simulink model "Australian14gen_following_inertia"  (R2017b)
settings: Solver=ode23tb  StartTime=0.0  StopTime=30  FixedStep=1e-3  RelTol=1e-5  AbsTol=1e-3  EnableMultiTasking=on
PreLoadFcn:
  | dataaustralian14gen
values from neighbouring files (symbols this model uses):
  alpha = -sys.follin.opt.alpha*1e8    [main_following.m]    (also in optimgains.mat = [-2447350365.29 -12566370614.4 -12566370614.4 -11730281347.7)
  bus_v = [ 101	15 ... (first row only)    [dataaustralian14gen.m]
  comp = [ 1	211	0	0 ... (first row only)    [dataaustralian14gen.m]
  dist = sys.follin.dist    [main_following.m]    (also in main_forming.m = sys.formin.dist)
  Exc = [ 101	0	 200	0.1	    13.25  2.5	 0	0       0       0       0       0 ... (first row only)    [dataaustralian14gen.m]
  FH = 13    [dataaustralian14gen.m]
  FI = 1    [dataaustralian14gen.m]
  FL = .1    (= 0.1)    [dataaustralian14gen.m]
  G_data = [ 101	333.3	15	3.6	0.14	1.1	0.65	0.25	8.5     0.25	0.05	0       0       0.25	0.2 	0 ... (first row only)    [dataaustralian14gen.m]
  KH = 120    [dataaustralian14gen.m]
  KI = 10    [dataaustralian14gen.m]
  KL = 10    [dataaustralian14gen.m]
  line = [ 102	217	0.0084	0.0667	0.817	330	1 ... (first row only)    [dataaustralian14gen.m]
  load_mag = load_case4    [dataaustralian14gen.m]
  p = p_case4    [dataaustralian14gen.m]
  PLL_Ki = 2    [dataaustralian14gen.m]
  PLL_Kp = 500    [dataaustralian14gen.m]
  PSSMODEL = 1    [dataaustralian14gen.m]
  trans = [ 1	101	102	15	330	333.3	12	12 ... (first row only)    [dataaustralian14gen.m]
undefined symbols (not defined in the file or in its folder): D1, Delta, sys
libraries: powerlib x353, Library x30, powerlib_meascontrol x15, sps_avr x10, powerlib_extras x4
(part 2 of 4)

== system Australian14gen_following_inertia/Dist206 ==
  Constant : Constant  Value=0
  Dist206 : Step  Time=dist.time  After=dist.inp(1)  SampleTime=0
  Gain : Gain  Gain=-1
  Mux : Mux  Inputs=2
  virtin : powerlib/Elements/Three-Phase Dynamic Load  NominalVoltage=[ 20e3 50 ]  ActiveReactivePowers=[0 0]  PositiveSequence=[1.01445 26.5635]  ExternalControl=on  NpNq="[0  0]"  TimeConstants="[0  0  0  0]"  MinimumVoltage=0.01  Tfilter=1e-1  LoadFlowParameters=[4 50000000 0 0 25000000]
      settings: SourceProductName=Simscape Power Systems  SourceProductBaseCode=PS
  A : PMIOPort  Port=1  Side=Right
  B : PMIOPort  Port=2  Side=Right
  C : PMIOPort  Port=3  Side=Right
  wires:
  Mux/1 -> Gain/1
  Gain/1 -> virtin/1
  Constant/1 -> Mux/2
  Dist206/1 -> Mux/1
  connections:
  B/RConn1 -- virtin/LConn2
  C/RConn1 -- virtin/LConn3
  A/RConn1 -- virtin/LConn1

== system Australian14gen_following_inertia/Dist212 ==
  Constant : Constant  Value=0
  Dist212 : Step  Time=dist.time  After=dist.inp(2)  SampleTime=0
  Gain : Gain  Gain=-1
  Mux : Mux  Inputs=2
  virtin : powerlib/Elements/Three-Phase Dynamic Load  NominalVoltage=[ 20e3 50 ]  ActiveReactivePowers=[0 0]  PositiveSequence=[1.01948 15.3995]  ExternalControl=on  NpNq="[0  0]"  TimeConstants="[0  0  0  0]"  MinimumVoltage=0.01  Tfilter=1e-1  LoadFlowParameters=[4 50000000 0 0 25000000]
      settings: SourceProductName=Simscape Power Systems  SourceProductBaseCode=PS
  A : PMIOPort  Port=1  Side=Right
  B : PMIOPort  Port=2  Side=Right
  C : PMIOPort  Port=3  Side=Right
  wires:
  Mux/1 -> Gain/1
  Gain/1 -> virtin/1
  Constant/1 -> Mux/2
  Dist212/1 -> Mux/1
  connections:
  B/RConn1 -- virtin/LConn2
  C/RConn1 -- virtin/LConn3
  A/RConn1 -- virtin/LConn1

== system Australian14gen_following_inertia/Dist307 ==
  Constant : Constant  Value=0
  Dist307 : Step  Time=dist.time  After=dist.inp(3)  SampleTime=0
  Gain : Gain  Gain=-1
  Mux : Mux  Inputs=2
  virtin : powerlib/Elements/Three-Phase Dynamic Load  NominalVoltage=[ 20e3 50 ]  ActiveReactivePowers=[0 0]  PositiveSequence=[1.01917 0.102657]  ExternalControl=on  NpNq="[0  0]"  TimeConstants="[0  0  0  0]"  MinimumVoltage=0.01  Tfilter=1e-1  LoadFlowParameters=[4 50000000 0 0 25000000]
      settings: SourceProductName=Simscape Power Systems  SourceProductBaseCode=PS
  A : PMIOPort  Port=1  Side=Right
  B : PMIOPort  Port=2  Side=Right
  C : PMIOPort  Port=3  Side=Right
  wires:
  Mux/1 -> Gain/1
  Gain/1 -> virtin/1
  Constant/1 -> Mux/2
  Dist307/1 -> Mux/1
  connections:
  B/RConn1 -- virtin/LConn2
  C/RConn1 -- virtin/LConn3
  A/RConn1 -- virtin/LConn1

== system Australian14gen_following_inertia/Dist410 ==
  Constant : Constant  Value=0
  Dist410 : Step  Time=dist.time  After=dist.inp(4)  SampleTime=0
  Gain : Gain  Gain=-1
  Mux : Mux  Inputs=2
  virtin : powerlib/Elements/Three-Phase Dynamic Load  NominalVoltage=[ 20e3 50 ]  ActiveReactivePowers=[0 0]  PositiveSequence=[0.580561 31.9916]  ExternalControl=on  NpNq="[0  0]"  TimeConstants="[0  0  0  0]"  MinimumVoltage=0.01  Tfilter=1e-1  LoadFlowParameters=[4 50000000 0 0 25000000]
      settings: SourceProductName=Simscape Power Systems  SourceProductBaseCode=PS
  A : PMIOPort  Port=1  Side=Right
  B : PMIOPort  Port=2  Side=Right
  C : PMIOPort  Port=3  Side=Right
  wires:
  Mux/1 -> Gain/1
  Gain/1 -> virtin/1
  Constant/1 -> Mux/2
  Dist410/1 -> Mux/1
  connections:
  B/RConn1 -- virtin/LConn2
  C/RConn1 -- virtin/LConn3
  A/RConn1 -- virtin/LConn1

== system Australian14gen_following_inertia/Dist411 ==
  Constant : Constant  Value=0
  Dist411 : Step  Time=dist.time  After=dist.inp(5)  SampleTime=0
  Gain : Gain  Gain=-1
  Mux : Mux  Inputs=2
  virtin : powerlib/Elements/Three-Phase Dynamic Load  NominalVoltage=[ 20e3 50 ]  ActiveReactivePowers=[0 0]  PositiveSequence=[1.01065 -3.89331]  ExternalControl=on  NpNq="[0  0]"  TimeConstants="[0  0  0  0]"  MinimumVoltage=0.01  Tfilter=1e-1  LoadFlowParameters=[4 50000000 0 0 25000000]
      settings: SourceProductName=Simscape Power Systems  SourceProductBaseCode=PS
  A : PMIOPort  Port=1  Side=Right
  B : PMIOPort  Port=2  Side=Right
  C : PMIOPort  Port=3  Side=Right
  wires:
  Mux/1 -> Gain/1
  Gain/1 -> virtin/1
  Constant/1 -> Mux/2
  Dist411/1 -> Mux/1
  connections:
  B/RConn1 -- virtin/LConn2
  C/RConn1 -- virtin/LConn3
  A/RConn1 -- virtin/LConn1

== system Australian14gen_following_inertia/Dist508 ==
  Constant : Constant  Value=0
  Dist508 : Step  Time=dist.time  After=dist.inp(6)  SampleTime=0
  Gain : Gain  Gain=-1
  Mux : Mux  Inputs=2
  virtin : powerlib/Elements/Three-Phase Dynamic Load  NominalVoltage=[ 20e3 50 ]  ActiveReactivePowers=[0 0]  PositiveSequence=[0.756642 -15.6575]  ExternalControl=on  NpNq="[0  0]"  TimeConstants="[0  0  0  0]"  MinimumVoltage=0.01  Tfilter=1e-1  LoadFlowParameters=[4 50000000 0 0 25000000]
      settings: SourceProductName=Simscape Power Systems  SourceProductBaseCode=PS
  A : PMIOPort  Port=1  Side=Right
  B : PMIOPort  Port=2  Side=Right
  C : PMIOPort  Port=3  Side=Right
  wires:
  Mux/1 -> Gain/1
  Gain/1 -> virtin/1
  Constant/1 -> Mux/2
  Dist508/1 -> Mux/1
  connections:
  B/RConn1 -- virtin/LConn2
  C/RConn1 -- virtin/LConn3
  A/RConn1 -- virtin/LConn1

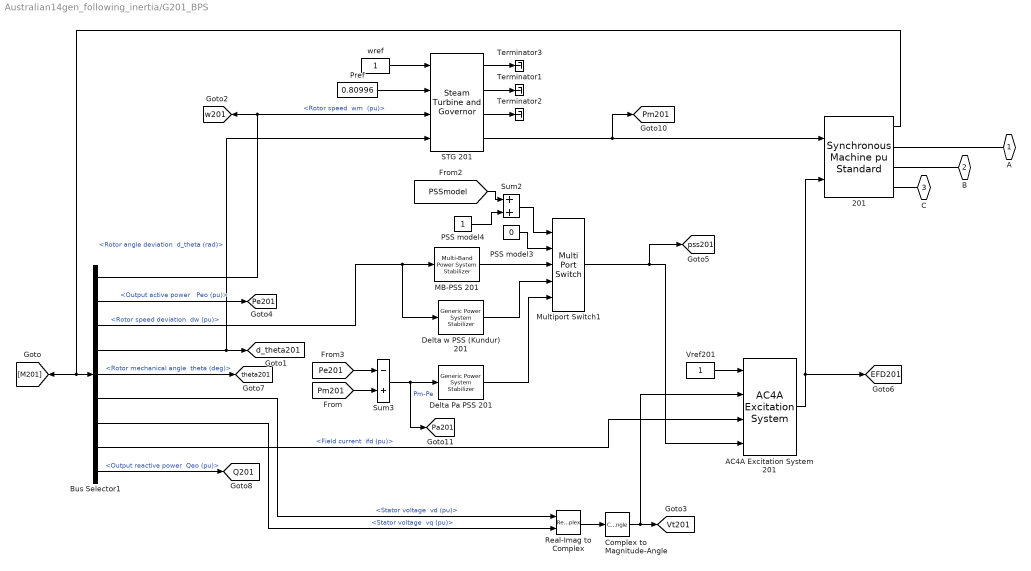
== system Australian14gen_following_inertia/G201_BPS ==
  201 : powerlib/Machines/Synchronous Machine pu Standard  PresetModel=No  MechanicalLoad=Mechanical power Pm  ShowDetailedParameters=on  RotorType=Round  Units=per unit standard parameters  MeasurementBus=off  NominalParameters="[G_data(2,2)*1e6  G_data(2,3)*1e3  50]"  Reactances1=[G_data(2,6),G_data(2,8),G_data(2,10),G_data(2,7),G_data(2,12),G_data(2,14),G_data(2,5)]  Reactances2=[G_data(2,6),G_data(2,8),G_data(2,10),G_data(2,7),G_data(2,14),G_data(2,5)]  dAxisTimeConstants=Open-circuit  qAxisTimeConstants=Open-circuit  TimeConstants1="[G_data(2,9)  G_data(2,11)  G_data(2,15)]"  TimeConstants2="[G_data(2,9), G_data(2,11), G_data(2,13),  G_data(2,15)]"  TimeConstants3="[  5.9  0.033  0.023  ]"  TimeConstants4=[ 8.0, 0.03, 0.3371, 0.0295 ]  TimeConstants5=[ 1.01, 0.053, 0.1 ]  TimeConstants6=[ 1.3201, 0.023, 1.0, 0.07 ]  TimeConstants7="[  1.01  0.053  0.051266  ]"  TimeConstants8=[ 1.3201, 0.0231, 0.3371, 0.0295 ]  StatorResistance=0  Mechanical="[ G_data(2,4) 0  4 ]"  PolePairs=4  InitialConditions=[0 -26.5731 0.812807 0.812807 0.812807 10.0885 -109.911 130.089 1.70153]  SetSaturation=off  Saturation=[0.6404,0.7127,0.8441,0.9214,0.9956,1.082,1.19,1.316,1.457;0.7,0.7698,0.8872,0.9466,0.9969,1.046,1.1,1.151,1.201]  LoadFlowParameters=[1 2160000000 20000 0 0]  TsPowergui=0  TsBlock=-1  IterativeModel=Forward Euler  IterativeDiscreteModel=Trapezoidal non iterative  BusType=PV  Pref=p(2,3)*1e6  Qref=0  Qmin=-inf  Qmax=inf  PLF=0  QLF=0
      settings: SourceProductName=Simscape Power Systems
  AC4A Excitation System 201 : sps_avr/AC4A Excitation System  Tr=Exc(2,2)  KaTa="[Exc(2,3)   Exc(2,4)]"  VIminmax=[-10 10]  VRminmax=[-4.53 5.64]  TbTc="[Exc(2,5)  Exc(2,6)]"  Kc=0  v0=[1 1.7015]  TsBlock=0
      settings: SourceProductName=Simscape Power Systems  SourceProductBaseCode=PS
  Bus Selector1 : BusSelector  OutputSignals="Mechanical.Rotor speed  wm  (pu),Output active power   Peo (pu),Mechanical.Rotor speed deviation  dw (pu),Mechanical.Rotor angle deviation  d_theta (rad),Mechanical.Rotor mechanical angle  theta (deg),dq0 components.Stator voltage  vd (pu),dq0 components.Stator voltage  vq (pu),dq0 components.Field current  ifd (pu),Output reactive power  Qeo (pu)"
  Complex to Magnitude-Angle : ComplexToMagnitudeAngle  Output=Magnitude
  Delta Pa PSS 201 : powerlib/Machines/Generic Power System Stabilizer  Tsensor=15e-3  K=2.5*1.25  Twashout=1  Tleadlag1=[60e-3 1]  Tleadlag2=[0 0]  VSlimits=[-0.15 0.15]  Vinit=0  Plot_On=off  MagdB_On=on  FreqRange=logspace(-2,2,500)
      settings: SourceProductName=Simscape Power Systems  SourceProductBaseCode=PS
  Delta w PSS (Kundur) 201 : powerlib/Machines/Generic Power System Stabilizer  Tsensor=15e-3  K=30  Twashout=10  Tleadlag1=[50e-3 20e-3]  Tleadlag2=[3 5.4]  VSlimits=[-0.15 0.15]  Vinit=0  Plot_On=off  MagdB_On=on  FreqRange=logspace(-2,2,500)
      settings: SourceProductName=Simscape Power Systems  SourceProductBaseCode=PS
  MB-PSS 201 : powerlib/Machines/Multi-Band Power System Stabilizer  OperationMode=Simplified settings  Kg=G  GL="[FL  KL]"  GI="[FI  KI]"  GH="[FH  KH]"  GLd=[66 66 9.4]  TcLF=[1.667 2 0 0 0 0 2 2.4 0 0 0 0 1 1]  GId=[66 66 47.6]  TcIF=[1 1 0.25 0.3 0 0 1 1 0.3 0.36 0 0 0 0]  GHd=[66 66 233]  TcHF="[0.01 0.012 0 0 0 0  0.012 0.0144 0 0 0 0 1 1]"  LIM=[.075 .15 .15 .15]  Plot_On=off  MagdB_On=off  FreqRange=logspace(-2,2,500)
      settings: SourceProductName=Simscape Power Systems  SourceProductBaseCode=PS
  Multiport Switch1 : MultiPortSwitch  Inputs=4  InputSameDT=on
  PSS model3 : Constant  Value=0
  PSS model4 : Constant
  Pref : Constant  Value=0.80996
  Real-Imag to Complex : RealImagToComplex
  STG 201 : powerlib/Machines/Steam Turbine and Governor  gentype=Tandem-compound (single mass)  reg1="[ 1  0.05    0 ]"  reg2="[ 0.001  0.15 ]"  reg3="[ -0.1  0.1  0  4.496 ]"  N=3000  turb1="[ 0  10   3.3   0.5   ]"  turb2="[   0   0.36    0.36   0.28   ]"  HA="[ 0.046  1.430  1.465   0.192 ]"  KA="[ 90.44  53.88  64.59   62.94  ]"  DA="[ 0.0115  0.3575  0.3663   0.0137  ]"  ini1=0.80996  ini2=[0.779316,-31.4247]
      settings: SourceProductName=Simscape Power Systems  SourceProductBaseCode=PS
  Sum2 : Sum  SaturateOnIntegerOverflow=on  InputSameDT=on  OutDataTypeStr=Inherit: Same as first input
  Sum3 : Sum  Inputs=-+  SaturateOnIntegerOverflow=on  InputSameDT=on  OutDataTypeStr=Inherit: Same as first input
  Terminator1 : Terminator
  Terminator2 : Terminator
  Terminator3 : Terminator
  Vref201 : Constant
  wref : Constant
  A : PMIOPort  Port=1  Side=Left
  B : PMIOPort  Port=2  Side=Left
  C : PMIOPort  Port=3  Side=Left
  tag scope: EFD201=global, Pa201=global, Pe201=global, Pm201=global, Q201=global, Vt201=global, d_theta201=global, pss201=global, theta201=global, w201=global
  wires:
  Bus Selector1/7 -> Real-Imag to Complex/2  "<Stator voltage  vq (pu)>"
  Bus Selector1/6 -> Real-Imag to Complex/1  "<Stator voltage  vd (pu)>"
  wref/1 -> STG 201/1
  Vref201/1 -> AC4A Excitation System 201/1
  Bus Selector1/4 -> STG 201/4, [d_theta201]  "<Rotor angle deviation  d_theta (rad)>"
  201/1 -> Bus Selector1/1, [M201]
  Bus Selector1/1 -> [w201], STG 201/3  "<Rotor speed  wm  (pu)>"
  Bus Selector1/3 -> Delta w PSS (Kundur) 201/1, MB-PSS 201/1  "<Rotor speed deviation  dw (pu)>"
  Real-Imag to Complex/1 -> Complex to Magnitude-Angle/1
  Complex to Magnitude-Angle/1 -> AC4A Excitation System 201/2, [Vt201]
  AC4A Excitation System 201/1 -> 201/2, [EFD201]
  Multiport Switch1/1 -> [pss201], AC4A Excitation System 201/4
  Bus Selector1/5 -> [theta201]  "<Rotor mechanical angle  theta (deg)>"
  Bus Selector1/2 -> [Pe201]  "<Output active power   Peo (pu)>"
  Bus Selector1/8 -> AC4A Excitation System 201/3  "<Field current  ifd (pu)>"
  Pref/1 -> STG 201/2
  STG 201/4 -> [Pm201], 201/1
  Bus Selector1/9 -> [Q201]  "<Output reactive power  Qeo (pu)>"
  PSS model4/1 -> Sum2/2
  Sum2/1 -> Multiport Switch1/1
  [PSSmodel] -> Sum2/1
  PSS model3/1 -> Multiport Switch1/2
  Sum3/1 -> [Pa201], Delta Pa PSS 201/1  "Pm-Pe"
  Delta Pa PSS 201/1 -> Multiport Switch1/5
  Delta w PSS (Kundur) 201/1 -> Multiport Switch1/4
  [Pm201] -> Sum3/2
  [Pe201] -> Sum3/1
  MB-PSS 201/1 -> Multiport Switch1/3
  STG 201/1 -> Terminator3/1
  STG 201/2 -> Terminator1/1
  STG 201/3 -> Terminator2/1
  connections:
  201/RConn1 -- A/RConn1
  201/RConn2 -- B/RConn1
  201/RConn3 -- C/RConn1

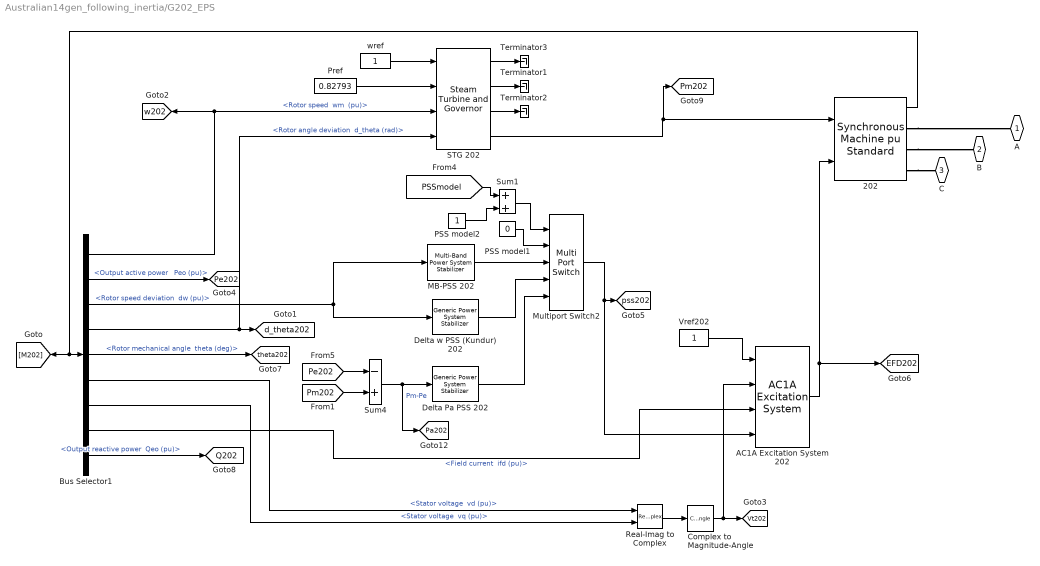
== system Australian14gen_following_inertia/G202_EPS ==
  202 : powerlib/Machines/Synchronous Machine pu Standard  PresetModel=No  MechanicalLoad=Mechanical power Pm  ShowDetailedParameters=on  RotorType=Round  Units=per unit standard parameters  MeasurementBus=off  NominalParameters="[G_data(3,2)*1e6  G_data(3,3)*1e3  50]"  Reactances1=[G_data(3,6),G_data(3,8),G_data(3,10),G_data(3,7),G_data(3,12), G_data(3,14),G_data(3,5)]  Reactances2=[G_data(3,6),G_data(3,8),G_data(3,10),G_data(3,7),G_data(3,12), G_data(3,14),G_data(3,5)]  dAxisTimeConstants=Open-circuit  qAxisTimeConstants=Open-circuit  TimeConstants1="[G_data(3,9)  G_data(3,11)  G_data(3,13) G_data(3,15)]"  TimeConstants2="[G_data(3,9)  G_data(3,11)  G_data(3,13) G_data(3,15)]"  TimeConstants3="[  5.9  0.033  0.023  ]"  TimeConstants4=[ 8.0, 0.03, 0.3371, 0.0295 ]  TimeConstants5=[ 1.01, 0.053, 0.1 ]  TimeConstants6=[ 1.3201, 0.023, 1.0, 0.07 ]  TimeConstants7="[  1.01  0.053  0.051266  ]"  TimeConstants8=[ 1.3201, 0.0231, 0.3371, 0.0295 ]  StatorResistance=0  Mechanical="[ G_data(3,4) 0  4 ]"  PolePairs=4  InitialConditions=[0 -26.5315 0.829135 0.829135 0.829135 4.08474 -115.915 124.085 2.03205]  SetSaturation=off  Saturation=[0.6404,0.7127,0.8441,0.9214,0.9956,1.082,1.19,1.316,1.457;0.7,0.7698,0.8872,0.9466,0.9969,1.046,1.1,1.151,1.201]  LoadFlowParameters=[1 1380000000 20000 0 0]  TsPowergui=0  TsBlock=-1  IterativeModel=Forward Euler  IterativeDiscreteModel=Trapezoidal non iterative  BusType=PV  Pref=p(3,3)*1e6  Qref=0  Qmin=-inf  Qmax=inf  PLF=0  QLF=0
      settings: SourceProductName=Simscape Power Systems
  AC1A Excitation System 202 : sps_avr/AC1A Excitation System  Tr=Exc(3,2)  KaTa="[Exc(3,3)   Exc(3,4)]"  VAminmax=[-14.5 14.5]  VRminmax=[-5.43 6.03]  KfTf="[Exc(3,9)  Exc(3,10)]"  TbTc="[Exc(3,5)  Exc(3,6)]"  KeTe="[Exc(3,7)  Exc(3,8)]"  Ve12=[4.18 3.14]  SeVe12=[0.10 0.03]  Kd=0.38  Kc=0.20  v0=[1 2.032]  TsBlock=0
      settings: SourceProductName=Simscape Power Systems  SourceProductBaseCode=PS
  Bus Selector1 : BusSelector  OutputSignals="Mechanical.Rotor speed  wm  (pu),Output active power   Peo (pu),Mechanical.Rotor speed deviation  dw (pu),Mechanical.Rotor angle deviation  d_theta (rad),Mechanical.Rotor mechanical angle  theta (deg),dq0 components.Stator voltage  vd (pu),dq0 components.Stator voltage  vq (pu),dq0 components.Field current  ifd (pu),Output reactive power  Qeo (pu)"
  Complex to Magnitude-Angle : ComplexToMagnitudeAngle  Output=Magnitude
  Delta Pa PSS 202 : powerlib/Machines/Generic Power System Stabilizer  Tsensor=15e-3  K=2.5*1.25  Twashout=1  Tleadlag1=[60e-3 1]  Tleadlag2=[0 0]  VSlimits=[-0.15 0.15]  Vinit=0  Plot_On=off  MagdB_On=on  FreqRange=logspace(-2,2,500)
      settings: SourceProductName=Simscape Power Systems  SourceProductBaseCode=PS
  Delta w PSS (Kundur) 202 : powerlib/Machines/Generic Power System Stabilizer  Tsensor=15e-3  K=30  Twashout=10  Tleadlag1=[50e-3 20e-3]  Tleadlag2=[3 5.4]  VSlimits=[-0.15 0.15]  Vinit=0  Plot_On=off  MagdB_On=on  FreqRange=logspace(-2,2,500)
      settings: SourceProductName=Simscape Power Systems  SourceProductBaseCode=PS
  MB-PSS 202 : powerlib/Machines/Multi-Band Power System Stabilizer  OperationMode=Simplified settings  Kg=G  GL="[FL  KL]"  GI="[FI  KI]"  GH="[FH  KH]"  GLd=[66 66 9.4]  TcLF=[1.667 2 0 0 0 0 2 2.4 0 0 0 0 1 1]  GId=[66 66 47.6]  TcIF=[1 1 0.25 0.3 0 0 1 1 0.3 0.36 0 0 0 0]  GHd=[66 66 233]  TcHF="[0.01 0.012 0 0 0 0  0.012 0.0144 0 0 0 0 1 1]"  LIM=[.075 .15 .15 .15]  Plot_On=off  MagdB_On=off  FreqRange=logspace(-2,2,500)
      settings: SourceProductName=Simscape Power Systems  SourceProductBaseCode=PS
  Multiport Switch2 : MultiPortSwitch  Inputs=4  InputSameDT=on
  PSS model1 : Constant  Value=0
  PSS model2 : Constant
  Pref : Constant  Value=0.82793
  Real-Imag to Complex : RealImagToComplex
  STG 202 : powerlib/Machines/Steam Turbine and Governor  gentype=Tandem-compound (single mass)  reg1="[ 1  0.05    0 ]"  reg2="[ 0.001  0.15 ]"  reg3="[ -0.1  0.1  0  4.496 ]"  N=3000  turb1="[ 0  10   3.3   0.5   ]"  turb2="[   0   0.36    0.36   0.28   ]"  HA="[ 0.046  1.430  1.465   0.192 ]"  KA="[ 90.44  53.88  64.59   62.94  ]"  DA="[ 0.0115  0.3575  0.3663   0.0137  ]"  ini1=0.82793  ini2=[0.779316,-31.4247]
      settings: SourceProductName=Simscape Power Systems  SourceProductBaseCode=PS
  Sum1 : Sum  SaturateOnIntegerOverflow=on  InputSameDT=on  OutDataTypeStr=Inherit: Same as first input
  Sum4 : Sum  Inputs=-+  SaturateOnIntegerOverflow=on  InputSameDT=on  OutDataTypeStr=Inherit: Same as first input
  Terminator1 : Terminator
  Terminator2 : Terminator
  Terminator3 : Terminator
  Vref202 : Constant
  wref : Constant
  A : PMIOPort  Port=1  Side=Left
  B : PMIOPort  Port=2  Side=Left
  C : PMIOPort  Port=3  Side=Left
  tag scope: EFD202=global, Pa202=global, Pe202=global, Pm202=global, Q202=global, Vt202=global, d_theta202=global, pss202=global, theta202=global, w202=global
  wires:
  Bus Selector1/7 -> Real-Imag to Complex/2  "<Stator voltage  vq (pu)>"
  Bus Selector1/6 -> Real-Imag to Complex/1  "<Stator voltage  vd (pu)>"
  wref/1 -> STG 202/1
  Vref202/1 -> AC1A Excitation System 202/1
  Bus Selector1/4 -> STG 202/4, [d_theta202]  "<Rotor angle deviation  d_theta (rad)>"
  202/1 -> [M202], Bus Selector1/1
  Bus Selector1/1 -> STG 202/3, [w202]  "<Rotor speed  wm  (pu)>"
  Bus Selector1/3 -> MB-PSS 202/1, Delta w PSS (Kundur) 202/1  "<Rotor speed deviation  dw (pu)>"
  Real-Imag to Complex/1 -> Complex to Magnitude-Angle/1
  Complex to Magnitude-Angle/1 -> AC1A Excitation System 202/2, [Vt202]
  AC1A Excitation System 202/1 -> 202/2, [EFD202]
  Multiport Switch2/1 -> AC1A Excitation System 202/4, [pss202]
  Bus Selector1/5 -> [theta202]  "<Rotor mechanical angle  theta (deg)>"
  Bus Selector1/2 -> [Pe202]  "<Output active power   Peo (pu)>"
  Bus Selector1/8 -> AC1A Excitation System 202/3  "<Field current  ifd (pu)>"
  Pref/1 -> STG 202/2
  STG 202/4 -> [Pm202], 202/1
  Bus Selector1/9 -> [Q202]  "<Output reactive power  Qeo (pu)>"
  PSS model2/1 -> Sum1/2
  Sum1/1 -> Multiport Switch2/1
  [PSSmodel] -> Sum1/1
  PSS model1/1 -> Multiport Switch2/2
  Sum4/1 -> [Pa202], Delta Pa PSS 202/1  "Pm-Pe"
  Delta Pa PSS 202/1 -> Multiport Switch2/5
  Delta w PSS (Kundur) 202/1 -> Multiport Switch2/4
  [Pm202] -> Sum4/2
  [Pe202] -> Sum4/1
  MB-PSS 202/1 -> Multiport Switch2/3
  STG 202/1 -> Terminator3/1
  STG 202/2 -> Terminator1/1
  STG 202/3 -> Terminator2/1
  connections:
  202/RConn1 -- A/RConn1
  202/RConn2 -- B/RConn1
  202/RConn3 -- C/RConn1

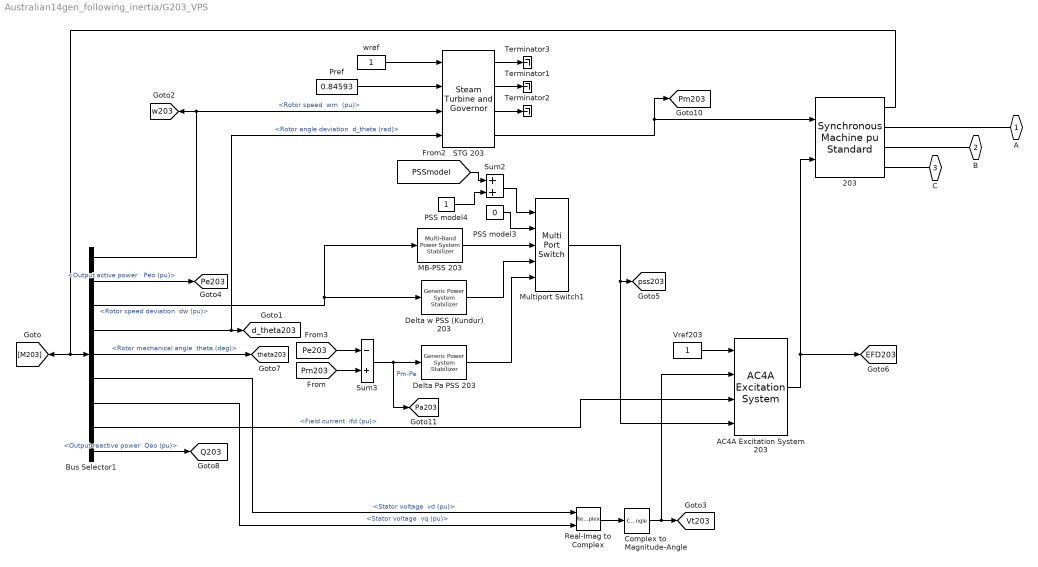
== system Australian14gen_following_inertia/G203_VPS ==
  203 : powerlib/Machines/Synchronous Machine pu Standard  PresetModel=No  MechanicalLoad=Mechanical power Pm  ShowDetailedParameters=on  RotorType=Round  Units=per unit standard parameters  MeasurementBus=off  NominalParameters="[G_data(4,2)*1E6  G_data(4,3)*1E3  50]"  Reactances1=[G_data(4,6),G_data(4,8),G_data(4,10),G_data(4,7),G_data(4,12),G_data(4,14),G_data(4,5)]  Reactances2=[G_data(4,6),G_data(4,8),G_data(4,10),G_data(4,7),G_data(4,14),G_data(4,5)]  dAxisTimeConstants=Open-circuit  qAxisTimeConstants=Open-circuit  TimeConstants1="[G_data(4,9)  G_data(4,11)  G_data(4,15)]"  TimeConstants2="[G_data(4,9)  G_data(4,11)  G_data(4,13)  G_data(4,15)]"  TimeConstants3="[  5.9  0.033  0.023  ]"  TimeConstants4=[ 8.0, 0.03, 0.3371, 0.0295 ]  TimeConstants5=[ 1.01, 0.053, 0.1 ]  TimeConstants6=[ 1.3201, 0.023, 1.0, 0.07 ]  TimeConstants7="[  1.01  0.053  0.051266  ]"  TimeConstants8=[ 1.3201, 0.0231, 0.3371, 0.0295 ]  StatorResistance=0  Mechanical="[ G_data(4,4) 0  4 ]"  PolePairs=4  InitialConditions=[0 -33.953 0.84594 0.84594 0.84594 0.941586 -119.058 120.942 2.16433]  SetSaturation=off  Saturation=[0.6404,0.7127,0.8441,0.9214,0.9956,1.082,1.19,1.316,1.457;0.7,0.7698,0.8872,0.9466,0.9969,1.046,1.1,1.151,1.201]  LoadFlowParameters=[1 1410000000 20000 0 0]  TsPowergui=0  TsBlock=-1  IterativeModel=Forward Euler  IterativeDiscreteModel=Trapezoidal non iterative  BusType=PV  Pref=p(4,3)*1e6  Qref=0  Qmin=-inf  Qmax=inf  PLF=0  QLF=0
      settings: SourceProductName=Simscape Power Systems
  AC4A Excitation System 203 : sps_avr/AC4A Excitation System  Tr=Exc(4,2)  KaTa="[Exc(4,3)   Exc(4,4)]"  VIminmax=[-10 10]  VRminmax=[-4.53 5.64]  TbTc="[Exc(4,5)  Exc(4,6)]"  Kc=0  v0=[1 2.1643]  TsBlock=0
      settings: SourceProductName=Simscape Power Systems  SourceProductBaseCode=PS
  Bus Selector1 : BusSelector  OutputSignals="Mechanical.Rotor speed  wm  (pu),Output active power   Peo (pu),Mechanical.Rotor speed deviation  dw (pu),Mechanical.Rotor angle deviation  d_theta (rad),Mechanical.Rotor mechanical angle  theta (deg),dq0 components.Stator voltage  vd (pu),dq0 components.Stator voltage  vq (pu),dq0 components.Field current  ifd (pu),Output reactive power  Qeo (pu)"
  Complex to Magnitude-Angle : ComplexToMagnitudeAngle  Output=Magnitude
  "Delta Pa PSS 203 " : powerlib/Machines/Generic Power System Stabilizer  Tsensor=15e-3  K=2.5*1.25  Twashout=1  Tleadlag1=[60e-3 1]  Tleadlag2=[0 0]  VSlimits=[-0.15 0.15]  Vinit=0  Plot_On=off  MagdB_On=on  FreqRange=logspace(-2,2,500)
      settings: SourceProductName=Simscape Power Systems  SourceProductBaseCode=PS
  "Delta w PSS (Kundur) 203 " : powerlib/Machines/Generic Power System Stabilizer  Tsensor=15e-3  K=30  Twashout=10  Tleadlag1=[50e-3 20e-3]  Tleadlag2=[3 5.4]  VSlimits=[-0.15 0.15]  Vinit=0  Plot_On=off  MagdB_On=on  FreqRange=logspace(-2,2,500)
      settings: SourceProductName=Simscape Power Systems  SourceProductBaseCode=PS
  "MB-PSS 203 " : powerlib/Machines/Multi-Band Power System Stabilizer  OperationMode=Simplified settings  Kg=G  GL="[FL  KL]"  GI="[FI  KI]"  GH="[FH  KH]"  GLd=[66 66 9.4]  TcLF=[1.667 2 0 0 0 0 2 2.4 0 0 0 0 1 1]  GId=[66 66 47.6]  TcIF=[1 1 0.25 0.3 0 0 1 1 0.3 0.36 0 0 0 0]  GHd=[66 66 233]  TcHF="[0.01 0.012 0 0 0 0  0.012 0.0144 0 0 0 0 1 1]"  LIM=[.075 .15 .15 .15]  Plot_On=off  MagdB_On=off  FreqRange=logspace(-2,2,500)
      settings: SourceProductName=Simscape Power Systems  SourceProductBaseCode=PS
  Multiport Switch1 : MultiPortSwitch  Inputs=4  InputSameDT=on
  PSS model3 : Constant  Value=0
  PSS model4 : Constant
  Pref : Constant  Value=0.84593
  Real-Imag to Complex : RealImagToComplex
  STG 203 : powerlib/Machines/Steam Turbine and Governor  gentype=Tandem-compound (single mass)  reg1="[ 1  0.05    0 ]"  reg2="[ 0.001  0.15 ]"  reg3="[ -0.1  0.1  0  4.496 ]"  N=3000  turb1="[ 0  10   3.3   0.5   ]"  turb2="[   0   0.36    0.36   0.28   ]"  HA="[ 0.046  1.430  1.465   0.192 ]"  KA="[ 90.44  53.88  64.59   62.94  ]"  DA="[ 0.0115  0.3575  0.3663   0.0137  ]"  ini1=0.84593  ini2=[0.779316,-31.4247]
      settings: SourceProductName=Simscape Power Systems  SourceProductBaseCode=PS
  Sum2 : Sum  SaturateOnIntegerOverflow=on  InputSameDT=on  OutDataTypeStr=Inherit: Same as first input
  Sum3 : Sum  Inputs=-+  SaturateOnIntegerOverflow=on  InputSameDT=on  OutDataTypeStr=Inherit: Same as first input
  Terminator1 : Terminator
  Terminator2 : Terminator
  Terminator3 : Terminator
  Vref203 : Constant
  wref : Constant
  A : PMIOPort  Port=1  Side=Left
  B : PMIOPort  Port=2  Side=Left
  C : PMIOPort  Port=3  Side=Left
  tag scope: EFD203=global, Pa203=global, Pe203=global, Pm203=global, Q203=global, Vt203=global, d_theta203=global, pss203=global, theta203=global, w203=global
  wires:
  Bus Selector1/7 -> Real-Imag to Complex/2  "<Stator voltage  vq (pu)>"
  Bus Selector1/6 -> Real-Imag to Complex/1  "<Stator voltage  vd (pu)>"
  wref/1 -> STG 203/1
  Vref203/1 -> AC4A Excitation System 203/1
  Bus Selector1/4 -> STG 203/4, [d_theta203]  "<Rotor angle deviation  d_theta (rad)>"
  203/1 -> [M203], Bus Selector1/1
  Bus Selector1/1 -> [w203], STG 203/3  "<Rotor speed  wm  (pu)>"
  Bus Selector1/3 -> "Delta w PSS (Kundur) 203 "/1, "MB-PSS 203 "/1  "<Rotor speed deviation  dw (pu)>"
  Real-Imag to Complex/1 -> Complex to Magnitude-Angle/1
  Complex to Magnitude-Angle/1 -> AC4A Excitation System 203/2, [Vt203]
  AC4A Excitation System 203/1 -> [EFD203], 203/2
  Multiport Switch1/1 -> AC4A Excitation System 203/4, [pss203]
  Bus Selector1/5 -> [theta203]  "<Rotor mechanical angle  theta (deg)>"
  Bus Selector1/2 -> [Pe203]  "<Output active power   Peo (pu)>"
  Bus Selector1/8 -> AC4A Excitation System 203/3  "<Field current  ifd (pu)>"
  Pref/1 -> STG 203/2
  STG 203/4 -> [Pm203], 203/1
  Bus Selector1/9 -> [Q203]  "<Output reactive power  Qeo (pu)>"
  PSS model4/1 -> Sum2/2
  Sum2/1 -> Multiport Switch1/1
  [PSSmodel] -> Sum2/1
  PSS model3/1 -> Multiport Switch1/2
  Sum3/1 -> [Pa203], "Delta Pa PSS 203 "/1  "Pm-Pe"
  "Delta Pa PSS 203 "/1 -> Multiport Switch1/5
  "Delta w PSS (Kundur) 203 "/1 -> Multiport Switch1/4
  [Pm203] -> Sum3/2
  [Pe203] -> Sum3/1
  "MB-PSS 203 "/1 -> Multiport Switch1/3
  STG 203/1 -> Terminator3/1
  STG 203/2 -> Terminator1/1
  STG 203/3 -> Terminator2/1
  connections:
  203/RConn1 -- A/RConn1
  203/RConn2 -- B/RConn1
  203/RConn3 -- C/RConn1

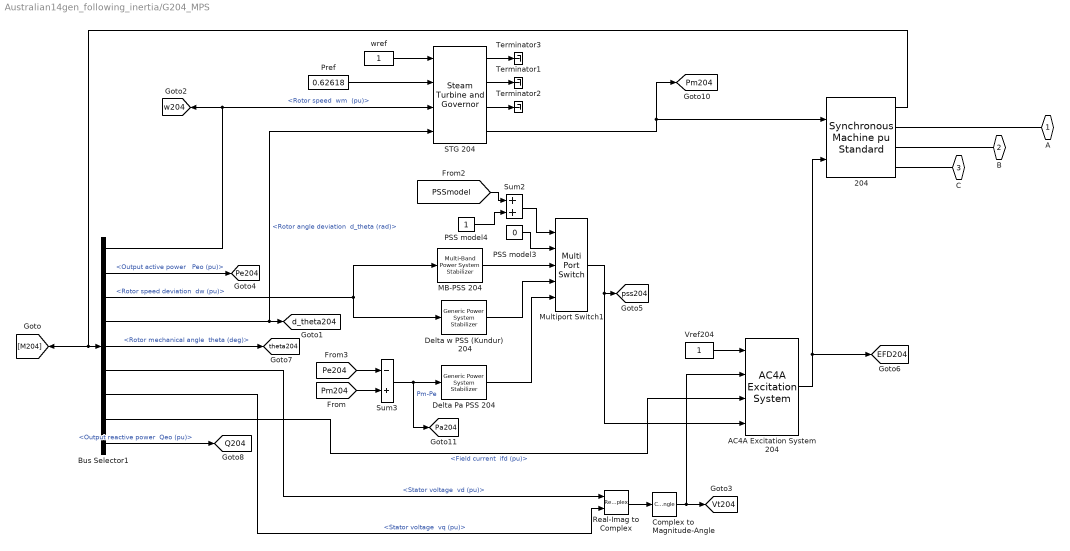
== system Australian14gen_following_inertia/G204_MPS ==
  204 : powerlib/Machines/Synchronous Machine pu Standard  PresetModel=No  MechanicalLoad=Mechanical power Pm  ShowDetailedParameters=on  RotorType=Round  Units=per unit standard parameters  MeasurementBus=off  NominalParameters="[G_data(5,2)*1E6  G_data(5,3)*1E3  50]"  Reactances1=[G_data(5,6),G_data(5,8),G_data(5,10),G_data(5,7),G_data(5,12),G_data(5,14),G_data(5,5)]  Reactances2=[G_data(5,6),G_data(5,8),G_data(5,10),G_data(5,7),G_data(5,12),G_data(5,14),G_data(5,5)]  dAxisTimeConstants=Open-circuit  qAxisTimeConstants=Open-circuit  TimeConstants1="[G_data(5,9)  G_data(5,11)  G_data(5,13) G_data(5,15)]"  TimeConstants2="[G_data(5,9)  G_data(5,11)  G_data(5,13) G_data(5,15)]"  TimeConstants3="[  5.9  0.033  0.023  ]"  TimeConstants4=[ 8.0, 0.03, 0.3371, 0.0295 ]  TimeConstants5=[ 1.01, 0.053, 0.1 ]  TimeConstants6=[ 1.3201, 0.023, 1.0, 0.07 ]  TimeConstants7="[  1.01  0.053  0.051266  ]"  TimeConstants8=[ 1.3201, 0.0231, 0.3371, 0.0295 ]  StatorResistance=0  Mechanical="[ G_data(5,4) 0  4 ]"  PolePairs=4  InitialConditions=[0 -37.6642 0.632347 0.632347 0.632347 8.00726 -111.993 128.007 1.40639]  SetSaturation=off  Saturation=[0.6404,0.7127,0.8441,0.9214,0.9956,1.082,1.19,1.316,1.457;0.7,0.7698,0.8872,0.9466,0.9969,1.046,1.1,1.151,1.201]  LoadFlowParameters=[2 1987000000 20000 0 0]  TsPowergui=0  TsBlock=-1  IterativeModel=Forward Euler  IterativeDiscreteModel=Trapezoidal non iterative  BusType=swing  Pref=p(5,3)*1e6  Qref=0  Qmin=-inf  Qmax=inf  PLF=0  QLF=0
      settings: SourceProductName=Simscape Power Systems
  AC4A Excitation System 204 : sps_avr/AC4A Excitation System  Tr=Exc(5,2)  KaTa="[Exc(5,3)   Exc(5,4)]"  VIminmax=[-10 10]  VRminmax=[-4.53 5.64]  TbTc="[Exc(5,5)  Exc(5,6)]"  Kc=0  v0=[1 1.4064]  TsBlock=0
      settings: SourceProductName=Simscape Power Systems  SourceProductBaseCode=PS
  Bus Selector1 : BusSelector  OutputSignals="Mechanical.Rotor speed  wm  (pu),Output active power   Peo (pu),Mechanical.Rotor speed deviation  dw (pu),Mechanical.Rotor angle deviation  d_theta (rad),Mechanical.Rotor mechanical angle  theta (deg),dq0 components.Stator voltage  vd (pu),dq0 components.Stator voltage  vq (pu),dq0 components.Field current  ifd (pu),Output reactive power  Qeo (pu)"
  Complex to Magnitude-Angle : ComplexToMagnitudeAngle  Output=Magnitude
  "Delta Pa PSS 204 " : powerlib/Machines/Generic Power System Stabilizer  Tsensor=15e-3  K=2.5*1.25  Twashout=1  Tleadlag1=[60e-3 1]  Tleadlag2=[0 0]  VSlimits=[-0.15 0.15]  Vinit=0  Plot_On=off  MagdB_On=on  FreqRange=logspace(-2,2,500)
      settings: SourceProductName=Simscape Power Systems  SourceProductBaseCode=PS
  Delta w PSS (Kundur)  204 : powerlib/Machines/Generic Power System Stabilizer  Tsensor=15e-3  K=30  Twashout=10  Tleadlag1=[50e-3 20e-3]  Tleadlag2=[3 5.4]  VSlimits=[-0.15 0.15]  Vinit=0  Plot_On=off  MagdB_On=on  FreqRange=logspace(-2,2,500)
      settings: SourceProductName=Simscape Power Systems  SourceProductBaseCode=PS
  "MB-PSS 204 " : powerlib/Machines/Multi-Band Power System Stabilizer  OperationMode=Simplified settings  Kg=G  GL="[FL  KL]"  GI="[FI  KI]"  GH="[FH  KH]"  GLd=[66 66 9.4]  TcLF=[1.667 2 0 0 0 0 2 2.4 0 0 0 0 1 1]  GId=[66 66 47.6]  TcIF=[1 1 0.25 0.3 0 0 1 1 0.3 0.36 0 0 0 0]  GHd=[66 66 233]  TcHF="[0.01 0.012 0 0 0 0  0.012 0.0144 0 0 0 0 1 1]"  LIM=[.075 .15 .15 .15]  Plot_On=off  MagdB_On=off  FreqRange=logspace(-2,2,500)
      settings: SourceProductName=Simscape Power Systems  SourceProductBaseCode=PS
  Multiport Switch1 : MultiPortSwitch  Inputs=4  InputSameDT=on
  PSS model3 : Constant  Value=0
  PSS model4 : Constant
  Pref : Constant  Value=0.62618
  Real-Imag to Complex : RealImagToComplex
  STG 204 : powerlib/Machines/Steam Turbine and Governor  gentype=Tandem-compound (single mass)  reg1="[ 1  0.05    0 ]"  reg2="[ 0.001  0.15 ]"  reg3="[ -0.1  0.1  0  4.496 ]"  N=3000  turb1="[ 0  10   3.3   0.5   ]"  turb2="[   0   0.36    0.36   0.28   ]"  HA="[ 0.046  1.430  1.465   0.192 ]"  KA="[ 90.44  53.88  64.59   62.94  ]"  DA="[ 0.0115  0.3575  0.3663   0.0137  ]"  ini1=0.62618  ini2=[0.779316,-31.4247]
      settings: SourceProductName=Simscape Power Systems  SourceProductBaseCode=PS
  Sum2 : Sum  SaturateOnIntegerOverflow=on  InputSameDT=on  OutDataTypeStr=Inherit: Same as first input
  Sum3 : Sum  Inputs=-+  SaturateOnIntegerOverflow=on  InputSameDT=on  OutDataTypeStr=Inherit: Same as first input
  Terminator1 : Terminator
  Terminator2 : Terminator
  Terminator3 : Terminator
  Vref204 : Constant
  wref : Constant
  A : PMIOPort  Port=1  Side=Left
  B : PMIOPort  Port=2  Side=Left
  C : PMIOPort  Port=3  Side=Left
  tag scope: EFD204=global, Pa204=global, Pe204=global, Pm204=global, Q204=global, Vt204=global, d_theta204=global, pss204=global, theta204=global, w204=global
  wires:
  Bus Selector1/7 -> Real-Imag to Complex/2  "<Stator voltage  vq (pu)>"
  Bus Selector1/6 -> Real-Imag to Complex/1  "<Stator voltage  vd (pu)>"
  wref/1 -> STG 204/1
  Vref204/1 -> AC4A Excitation System 204/1
  Bus Selector1/4 -> STG 204/4, [d_theta204]  "<Rotor angle deviation  d_theta (rad)>"
  204/1 -> [M204], Bus Selector1/1
  Bus Selector1/1 -> [w204], STG 204/3  "<Rotor speed  wm  (pu)>"
  Bus Selector1/3 -> Delta w PSS (Kundur)  204/1, "MB-PSS 204 "/1  "<Rotor speed deviation  dw (pu)>"
  Real-Imag to Complex/1 -> Complex to Magnitude-Angle/1
  Complex to Magnitude-Angle/1 -> AC4A Excitation System 204/2, [Vt204]
  AC4A Excitation System 204/1 -> [EFD204], 204/2
  Multiport Switch1/1 -> AC4A Excitation System 204/4, [pss204]
  Bus Selector1/5 -> [theta204]  "<Rotor mechanical angle  theta (deg)>"
  Bus Selector1/2 -> [Pe204]  "<Output active power   Peo (pu)>"
  Bus Selector1/8 -> AC4A Excitation System 204/3  "<Field current  ifd (pu)>"
  Bus Selector1/9 -> [Q204]  "<Output reactive power  Qeo (pu)>"
  Pref/1 -> STG 204/2
  STG 204/4 -> [Pm204], 204/1
  PSS model4/1 -> Sum2/2
  Sum2/1 -> Multiport Switch1/1
  [PSSmodel] -> Sum2/1
  PSS model3/1 -> Multiport Switch1/2
  Sum3/1 -> [Pa204], "Delta Pa PSS 204 "/1  "Pm-Pe"
  "Delta Pa PSS 204 "/1 -> Multiport Switch1/5
  Delta w PSS (Kundur)  204/1 -> Multiport Switch1/4
  [Pm204] -> Sum3/2
  [Pe204] -> Sum3/1
  "MB-PSS 204 "/1 -> Multiport Switch1/3
  STG 204/1 -> Terminator3/1
  STG 204/2 -> Terminator1/1
  STG 204/3 -> Terminator2/1
  connections:
  204/RConn1 -- A/RConn1
  204/RConn2 -- B/RConn1
  204/RConn3 -- C/RConn1

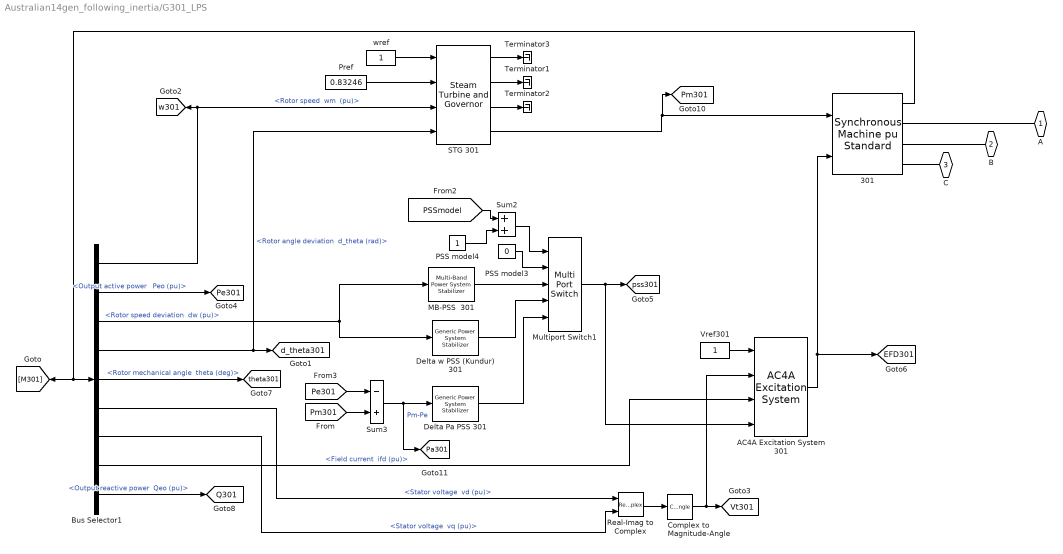
== system Australian14gen_following_inertia/G301_LPS ==
  301 : powerlib/Machines/Synchronous Machine pu Standard  PresetModel=No  MechanicalLoad=Mechanical power Pm  ShowDetailedParameters=on  RotorType=Round  Units=per unit standard parameters  MeasurementBus=off  NominalParameters="[G_data(6,2)*1E6  G_data(6,3)*1E3  50]"  Reactances1=[G_data(6,6),G_data(6,8),G_data(6,10),G_data(6,7),G_data(6,12),G_data(6,14),G_data(6,5)]  Reactances2=[G_data(6,6),G_data(6,8),G_data(6,10),G_data(6,7),G_data(6,12),G_data(6,14),G_data(6,5)]  dAxisTimeConstants=Open-circuit  qAxisTimeConstants=Open-circuit  TimeConstants1="[G_data(6,9)  G_data(6,11)  G_data(6,13)  G_data(6,15)]"  TimeConstants2="[G_data(6,9)  G_data(6,11)  G_data(6,13)  G_data(6,15)]"  TimeConstants3="[  5.9  0.033  0.023  ]"  TimeConstants4=[ 8.0, 0.03, 0.3371, 0.0295 ]  TimeConstants5=[ 1.01, 0.053, 0.1 ]  TimeConstants6=[ 1.3201, 0.023, 1.0, 0.07 ]  TimeConstants7="[  1.01  0.053  0.051266  ]"  TimeConstants8=[ 1.3201, 0.0231, 0.3371, 0.0295 ]  StatorResistance=0  Mechanical="[ G_data(6,4) 0  4 ]"  PolePairs=4  InitialConditions=[0 -46.5414 0.832459 0.832459 0.832459 -7.83521 -127.835 112.165 2.37871]  SetSaturation=off  Saturation=[0.6404,0.7127,0.8441,0.9214,0.9956,1.082,1.19,1.316,1.457;0.7,0.7698,0.8872,0.9466,0.9969,1.046,1.1,1.151,1.201]  LoadFlowParameters=[1 3330000000 20000 0 0]  TsPowergui=0  TsBlock=-1  IterativeModel=Forward Euler  IterativeDiscreteModel=Trapezoidal non iterative  BusType=PV  Pref=p(6,3)*1e6  Qref=0  Qmin=-inf  Qmax=inf  PLF=0  QLF=0
      settings: SourceProductName=Simscape Power Systems
  AC4A Excitation System 301 : sps_avr/AC4A Excitation System  Tr=Exc(6,2)  KaTa="[Exc(6,3)   Exc(6,4)]"  VIminmax=[-10 10]  VRminmax=[-4.53 5.64]  TbTc="[Exc(6,5)  Exc(6,6)]"  Kc=0  v0=[1 2.3787]  TsBlock=0
      settings: SourceProductName=Simscape Power Systems  SourceProductBaseCode=PS
  Bus Selector1 : BusSelector  OutputSignals="Mechanical.Rotor speed  wm  (pu),Output active power   Peo (pu),Mechanical.Rotor speed deviation  dw (pu),Mechanical.Rotor angle deviation  d_theta (rad),Mechanical.Rotor mechanical angle  theta (deg),dq0 components.Stator voltage  vd (pu),dq0 components.Stator voltage  vq (pu),dq0 components.Field current  ifd (pu),Output reactive power  Qeo (pu)"
  Complex to Magnitude-Angle : ComplexToMagnitudeAngle  Output=Magnitude
  "Delta Pa PSS 301 " : powerlib/Machines/Generic Power System Stabilizer  Tsensor=15e-3  K=2.5*1.25  Twashout=1  Tleadlag1=[60e-3 1]  Tleadlag2=[0 0]  VSlimits=[-0.15 0.15]  Vinit=0  Plot_On=off  MagdB_On=on  FreqRange=logspace(-2,2,500)
      settings: SourceProductName=Simscape Power Systems  SourceProductBaseCode=PS
  "Delta w PSS (Kundur) 301 " : powerlib/Machines/Generic Power System Stabilizer  Tsensor=15e-3  K=30  Twashout=10  Tleadlag1=[50e-3 20e-3]  Tleadlag2=[3 5.4]  VSlimits=[-0.15 0.15]  Vinit=0  Plot_On=off  MagdB_On=on  FreqRange=logspace(-2,2,500)
      settings: SourceProductName=Simscape Power Systems  SourceProductBaseCode=PS
  MB-PSS  301 : powerlib/Machines/Multi-Band Power System Stabilizer  OperationMode=Simplified settings  Kg=G  GL="[FL  KL]"  GI="[FI  KI]"  GH="[FH  KH]"  GLd=[66 66 9.4]  TcLF=[1.667 2 0 0 0 0 2 2.4 0 0 0 0 1 1]  GId=[66 66 47.6]  TcIF=[1 1 0.25 0.3 0 0 1 1 0.3 0.36 0 0 0 0]  GHd=[66 66 233]  TcHF="[0.01 0.012 0 0 0 0  0.012 0.0144 0 0 0 0 1 1]"  LIM=[.075 .15 .15 .15]  Plot_On=off  MagdB_On=off  FreqRange=logspace(-2,2,500)
      settings: SourceProductName=Simscape Power Systems  SourceProductBaseCode=PS
  Multiport Switch1 : MultiPortSwitch  Inputs=4  InputSameDT=on
  PSS model3 : Constant  Value=0
  PSS model4 : Constant
  Pref : Constant  Value=0.83246
  Real-Imag to Complex : RealImagToComplex
  STG 301 : powerlib/Machines/Steam Turbine and Governor  gentype=Tandem-compound (single mass)  reg1="[ 1  0.05    0 ]"  reg2="[ 0.001  0.15 ]"  reg3="[ -0.1  0.1  0  4.496 ]"  N=3000  turb1="[ 0  10   3.3   0.5   ]"  turb2="[   0   0.36    0.36   0.28   ]"  HA="[ 0.046  1.430  1.465   0.192 ]"  KA="[ 90.44  53.88  64.59   62.94  ]"  DA="[ 0.0115  0.3575  0.3663   0.0137  ]"  ini1=0.83246  ini2=[0.779316,-31.4247]
      settings: SourceProductName=Simscape Power Systems  SourceProductBaseCode=PS
  Sum2 : Sum  SaturateOnIntegerOverflow=on  InputSameDT=on  OutDataTypeStr=Inherit: Same as first input
  Sum3 : Sum  Inputs=-+  SaturateOnIntegerOverflow=on  InputSameDT=on  OutDataTypeStr=Inherit: Same as first input
  Terminator1 : Terminator
  Terminator2 : Terminator
  Terminator3 : Terminator
  Vref301 : Constant
  wref : Constant
  A : PMIOPort  Port=1  Side=Left
  B : PMIOPort  Port=2  Side=Left
  C : PMIOPort  Port=3  Side=Left
  tag scope: EFD301=global, Pa301=global, Pe301=global, Pm301=global, Q301=global, Vt301=global, d_theta301=global, pss301=global, theta301=global, w301=global
  wires:
  Bus Selector1/7 -> Real-Imag to Complex/2  "<Stator voltage  vq (pu)>"
  Bus Selector1/6 -> Real-Imag to Complex/1  "<Stator voltage  vd (pu)>"
  wref/1 -> STG 301/1
  Vref301/1 -> AC4A Excitation System 301/1
  Bus Selector1/4 -> [d_theta301], STG 301/4  "<Rotor angle deviation  d_theta (rad)>"
  301/1 -> Bus Selector1/1, [M301]
  Bus Selector1/1 -> [w301], STG 301/3  "<Rotor speed  wm  (pu)>"
  Bus Selector1/3 -> "Delta w PSS (Kundur) 301 "/1, MB-PSS  301/1  "<Rotor speed deviation  dw (pu)>"
  Real-Imag to Complex/1 -> Complex to Magnitude-Angle/1
  Complex to Magnitude-Angle/1 -> AC4A Excitation System 301/2, [Vt301]
  AC4A Excitation System 301/1 -> 301/2, [EFD301]
  Multiport Switch1/1 -> AC4A Excitation System 301/4, [pss301]
  Bus Selector1/5 -> [theta301]  "<Rotor mechanical angle  theta (deg)>"
  Bus Selector1/2 -> [Pe301]  "<Output active power   Peo (pu)>"
  Bus Selector1/8 -> AC4A Excitation System 301/3  "<Field current  ifd (pu)>"
  STG 301/4 -> [Pm301], 301/1
  Pref/1 -> STG 301/2
  Bus Selector1/9 -> [Q301]  "<Output reactive power  Qeo (pu)>"
  PSS model4/1 -> Sum2/2
  Sum2/1 -> Multiport Switch1/1
  [PSSmodel] -> Sum2/1
  PSS model3/1 -> Multiport Switch1/2
  Sum3/1 -> [Pa301], "Delta Pa PSS 301 "/1  "Pm-Pe"
  "Delta Pa PSS 301 "/1 -> Multiport Switch1/5
  "Delta w PSS (Kundur) 301 "/1 -> Multiport Switch1/4
  [Pm301] -> Sum3/2
  [Pe301] -> Sum3/1
  MB-PSS  301/1 -> Multiport Switch1/3
  STG 301/1 -> Terminator3/1
  STG 301/2 -> Terminator1/1
  STG 301/3 -> Terminator2/1
  connections:
  301/RConn1 -- A/RConn1
  301/RConn2 -- B/RConn1
  301/RConn3 -- C/RConn1

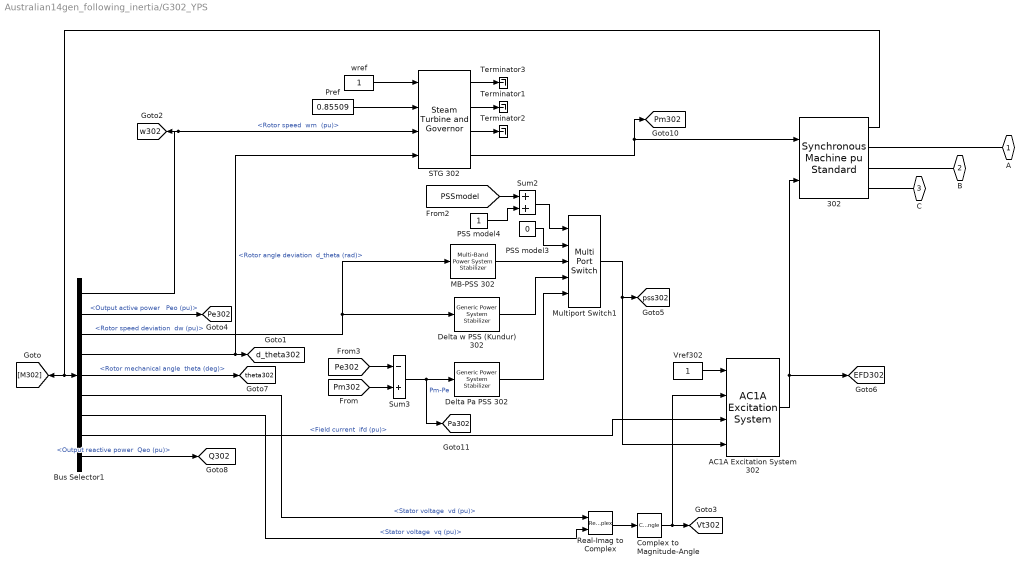
== system Australian14gen_following_inertia/G302_YPS ==
  302 : powerlib/Machines/Synchronous Machine pu Standard  PresetModel=No  MechanicalLoad=Mechanical power Pm  ShowDetailedParameters=on  RotorType=Round  Units=per unit standard parameters  MeasurementBus=off  NominalParameters="[G_data(7,2)*1E6  G_data(7,3)*1E3  50]"  Reactances1=[G_data(7,6),G_data(7,8),G_data(7,10),G_data(7,7),G_data(7,12),G_data(7,14),G_data(7,5)]  Reactances2=[G_data(7,6),G_data(7,8),G_data(7,10),G_data(7,7),G_data(7,12),G_data(7,14),G_data(7,5)]  dAxisTimeConstants=Open-circuit  qAxisTimeConstants=Open-circuit  TimeConstants1="[G_data(7,9)  G_data(7,11)  G_data(7,13)  G_data(7,15)]"  TimeConstants2="[G_data(7,9)  G_data(7,11)  G_data(7,13)  G_data(7,15)]"  TimeConstants3="[  5.9  0.033  0.023  ]"  TimeConstants4=[ 8.0, 0.03, 0.3371, 0.0295 ]  TimeConstants5=[ 1.01, 0.053, 0.1 ]  TimeConstants6=[ 1.3201, 0.023, 1.0, 0.07 ]  TimeConstants7="[  1.01  0.053  0.051266  ]"  TimeConstants8=[ 1.3201, 0.0231, 0.3371, 0.0295 ]  StatorResistance=0  Mechanical="[ G_data(7,4) 0  4 ]"  PolePairs=4  InitialConditions=[0 -51.3246 0.855776 0.855776 0.855776 -19.0246 -139.025 100.975 2.01459]  SetSaturation=off  Saturation=[0.6404,0.7127,0.8441,0.9214,0.9956,1.082,1.19,1.316,1.457;0.7,0.7698,0.8872,0.9466,0.9969,1.046,1.1,1.151,1.201]  LoadFlowParameters=[1 760000000 20000 0 0]  TsPowergui=0  TsBlock=-1  IterativeModel=Forward Euler  IterativeDiscreteModel=Trapezoidal non iterative  BusType=PV  Pref=p(7,3)*1e6  Qref=0  Qmin=-inf  Qmax=inf  PLF=0  QLF=0
      settings: SourceProductName=Simscape Power Systems
  AC1A Excitation System 302 : sps_avr/AC1A Excitation System  Tr=Exc(7,2)  KaTa="[Exc(7,3)   Exc(7,4)]"  VAminmax=[-14.5 14.5]  VRminmax=[-5.43 6.03]  KfTf="[Exc(7,9)  Exc(7,10)]"  TbTc="[Exc(7,5)  Exc(7,6)]"  KeTe="[Exc(7,7)  Exc(7,8)]"  Ve12=[4.18 3.14]  SeVe12=[0.10 0.03]  Kd=0.38  Kc=0.20  v0=[1 2.0146]  TsBlock=0
      settings: SourceProductName=Simscape Power Systems  SourceProductBaseCode=PS
  Bus Selector1 : BusSelector  OutputSignals="Mechanical.Rotor speed  wm  (pu),Output active power   Peo (pu),Mechanical.Rotor speed deviation  dw (pu),Mechanical.Rotor angle deviation  d_theta (rad),Mechanical.Rotor mechanical angle  theta (deg),dq0 components.Stator voltage  vd (pu),dq0 components.Stator voltage  vq (pu),dq0 components.Field current  ifd (pu),Output reactive power  Qeo (pu)"
  Complex to Magnitude-Angle : ComplexToMagnitudeAngle  Output=Magnitude
  Delta Pa PSS 302 : powerlib/Machines/Generic Power System Stabilizer  Tsensor=15e-3  K=2.5*1.25  Twashout=1  Tleadlag1=[60e-3 1]  Tleadlag2=[0 0]  VSlimits=[-0.15 0.15]  Vinit=0  Plot_On=off  MagdB_On=on  FreqRange=logspace(-2,2,500)
      settings: SourceProductName=Simscape Power Systems  SourceProductBaseCode=PS
  Delta w PSS (Kundur) 302 : powerlib/Machines/Generic Power System Stabilizer  Tsensor=15e-3  K=30  Twashout=10  Tleadlag1=[50e-3 20e-3]  Tleadlag2=[3 5.4]  VSlimits=[-0.15 0.15]  Vinit=0  Plot_On=off  MagdB_On=on  FreqRange=logspace(-2,2,500)
      settings: SourceProductName=Simscape Power Systems  SourceProductBaseCode=PS
  "MB-PSS 302 " : powerlib/Machines/Multi-Band Power System Stabilizer  OperationMode=Simplified settings  Kg=G  GL="[FL  KL]"  GI="[FI  KI]"  GH="[FH  KH]"  GLd=[66 66 9.4]  TcLF=[1.667 2 0 0 0 0 2 2.4 0 0 0 0 1 1]  GId=[66 66 47.6]  TcIF=[1 1 0.25 0.3 0 0 1 1 0.3 0.36 0 0 0 0]  GHd=[66 66 233]  TcHF="[0.01 0.012 0 0 0 0  0.012 0.0144 0 0 0 0 1 1]"  LIM=[.075 .15 .15 .15]  Plot_On=off  MagdB_On=off  FreqRange=logspace(-2,2,500)
      settings: SourceProductName=Simscape Power Systems  SourceProductBaseCode=PS
  Multiport Switch1 : MultiPortSwitch  Inputs=4  InputSameDT=on
  PSS model3 : Constant  Value=0
  PSS model4 : Constant
  Pref : Constant  Value=0.85509
  Real-Imag to Complex : RealImagToComplex
  STG 302 : powerlib/Machines/Steam Turbine and Governor  gentype=Tandem-compound (single mass)  reg1="[ 1  0.05    0 ]"  reg2="[ 0.001  0.15 ]"  reg3="[ -0.1  0.1  0  4.496 ]"  N=3000  turb1="[ 0  10   3.3   0.5   ]"  turb2="[   0   0.36    0.36   0.28   ]"  HA="[ 0.046  1.430  1.465   0.192 ]"  KA="[ 90.44  53.88  64.59   62.94  ]"  DA="[ 0.0115  0.3575  0.3663   0.0137  ]"  ini1=0.85509  ini2=[0.779316,-31.4247]
      settings: SourceProductName=Simscape Power Systems  SourceProductBaseCode=PS
  Sum2 : Sum  SaturateOnIntegerOverflow=on  InputSameDT=on  OutDataTypeStr=Inherit: Same as first input
  Sum3 : Sum  Inputs=-+  SaturateOnIntegerOverflow=on  InputSameDT=on  OutDataTypeStr=Inherit: Same as first input
  Terminator1 : Terminator
  Terminator2 : Terminator
  Terminator3 : Terminator
  Vref302 : Constant
  wref : Constant
  A : PMIOPort  Port=1  Side=Left
  B : PMIOPort  Port=2  Side=Left
  C : PMIOPort  Port=3  Side=Left
  tag scope: EFD302=global, Pa302=global, Pe302=global, Pm302=global, Q302=global, Vt302=global, d_theta302=global, pss302=global, theta302=global, w302=global
  wires:
  Bus Selector1/7 -> Real-Imag to Complex/2  "<Stator voltage  vq (pu)>"
  Bus Selector1/6 -> Real-Imag to Complex/1  "<Stator voltage  vd (pu)>"
  wref/1 -> STG 302/1
  Vref302/1 -> AC1A Excitation System 302/1
  Bus Selector1/4 -> STG 302/4, [d_theta302]  "<Rotor angle deviation  d_theta (rad)>"
  302/1 -> Bus Selector1/1, [M302]
  Bus Selector1/1 -> [w302], STG 302/3  "<Rotor speed  wm  (pu)>"
  Bus Selector1/3 -> Delta w PSS (Kundur) 302/1, "MB-PSS 302 "/1  "<Rotor speed deviation  dw (pu)>"
  Real-Imag to Complex/1 -> Complex to Magnitude-Angle/1
  Complex to Magnitude-Angle/1 -> AC1A Excitation System 302/2, [Vt302]
  AC1A Excitation System 302/1 -> 302/2, [EFD302]
  Multiport Switch1/1 -> AC1A Excitation System 302/4, [pss302]
  Bus Selector1/5 -> [theta302]  "<Rotor mechanical angle  theta (deg)>"
  Bus Selector1/2 -> [Pe302]  "<Output active power   Peo (pu)>"
  Bus Selector1/8 -> AC1A Excitation System 302/3  "<Field current  ifd (pu)>"
  Pref/1 -> STG 302/2
  STG 302/4 -> [Pm302], 302/1
  Bus Selector1/9 -> [Q302]  "<Output reactive power  Qeo (pu)>"
  PSS model4/1 -> Sum2/2
  Sum2/1 -> Multiport Switch1/1
  [PSSmodel] -> Sum2/1
  PSS model3/1 -> Multiport Switch1/2
  Sum3/1 -> [Pa302], Delta Pa PSS 302/1  "Pm-Pe"
  Delta Pa PSS 302/1 -> Multiport Switch1/5
  Delta w PSS (Kundur) 302/1 -> Multiport Switch1/4
  [Pm302] -> Sum3/2
  [Pe302] -> Sum3/1
  "MB-PSS 302 "/1 -> Multiport Switch1/3
  STG 302/1 -> Terminator3/1
  STG 302/2 -> Terminator1/1
  STG 302/3 -> Terminator2/1
  connections:
  302/RConn1 -- A/RConn1
  302/RConn2 -- B/RConn1
  302/RConn3 -- C/RConn1
